simulink model "desc_fcns_ex711"  (R2025b)
settings: Solver=VariableStepAuto  StartTime=0.0  StopTime=50  RelTol=1e-3
settings Model: Creator=Predrag  LastModifiedBy=Predrag

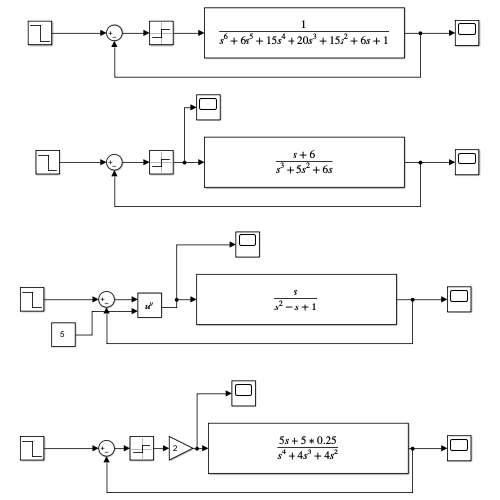
[thumbnail: Simulink's stored preview of the top-level diagram]
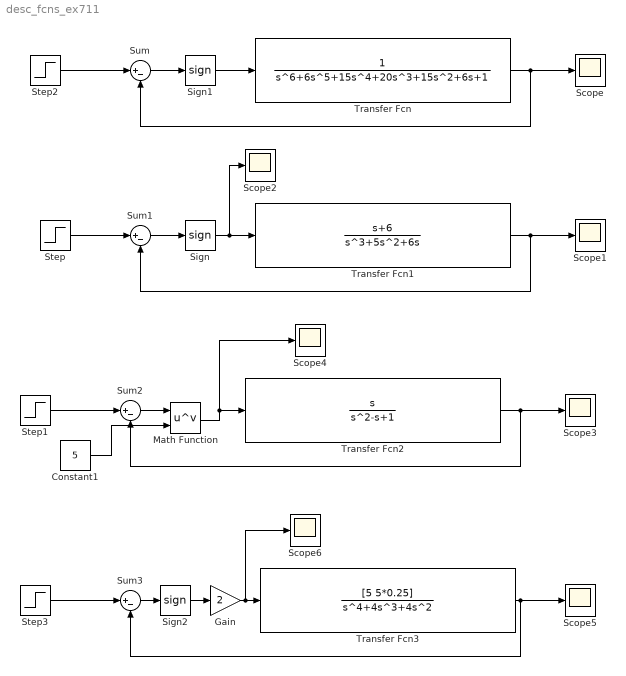
== system desc_fcns_ex711 ==
  Constant1 : Constant  Value=5
  Gain : Gain  Gain=2
  Math Function : Math  Operator=pow
  Scope{,1..6} (7 alike) : Scope
      Scope settings: ActiveDisplayYMinimum=-1  ActiveDisplayYMaximum=1
      Scope1 settings: ActiveDisplayYMinimum=-0.38866561213341477  ActiveDisplayYMaximum=1.399807651464674
      Scope2 settings: ActiveDisplayYMinimum=-2.4166666666666674  ActiveDisplayYMaximum=21.750000000000011  DataLoggingVariableName=ScopeData2
      Scope3 settings: ActiveDisplayYMinimum=-2.4166666666666674  ActiveDisplayYMaximum=21.750000000000011  DataLoggingVariableName=ScopeData3
      Scope4 settings: ActiveDisplayYMinimum=-2.4166666666666674  ActiveDisplayYMaximum=21.750000000000011  DataLoggingVariableName=ScopeData4
      Scope5 settings: ActiveDisplayYMinimum=-2.4166666666666674  ActiveDisplayYMaximum=21.750000000000011  DataLoggingVariableName=ScopeData5
      Scope6 settings: ActiveDisplayYMinimum=-2.4166666666666674  ActiveDisplayYMaximum=21.750000000000011  DataLoggingVariableName=ScopeData6
  Sign : Signum
  Sign1 : Signum
  Sign2 : Signum
  Step{,1..3} (4 alike) : Step  Time=3  Before=1  After=0  SampleTime=0
  Sum{,1..3} (4 alike) : Sum  Inputs=|+-
  Transfer Fcn : TransferFcn  Denominator=[1 6 15 20 15 6 1]
  Transfer Fcn1 : TransferFcn  Numerator=[1 6]  Denominator=[1 5 6 0]
  Transfer Fcn2 : TransferFcn  Numerator=[1 0]  Denominator=[1 -1 1]
  Transfer Fcn3 : TransferFcn  Numerator=[5 5*0.25]  Denominator=[1 4 4 0 0]
  wires:
  Transfer Fcn/1 -> Sum/2, Scope/1
  Sum/1 -> Sign1/1
  Sign1/1 -> Transfer Fcn/1
  Step2/1 -> Sum/1
  Sign/1 -> Scope2/1, Transfer Fcn1/1
  Sum1/1 -> Sign/1
  Transfer Fcn1/1 -> Scope1/1, Sum1/2
  Transfer Fcn2/1 -> Sum2/2, Scope3/1
  Sum2/1 -> Math Function/1
  Math Function/1 -> Transfer Fcn2/1, Scope4/1
  Step1/1 -> Sum2/1
  Constant1/1 -> Math Function/2
  Step/1 -> Sum1/1
  Step3/1 -> Sum3/1
  Sum3/1 -> Sign2/1
  Transfer Fcn3/1 -> Scope5/1, Sum3/2
  Sign2/1 -> Gain/1
  Gain/1 -> Scope6/1, Transfer Fcn3/1
